simulink model "sensorLib"  (R2020b)
settings: Solver=FixedStepAuto  StartTime=0.0  StopTime=10.0  FixedStep=Ts  RelTol=1e-3
undefined symbols (not defined in the file or in its folder): Sensors, States, Ts
libraries: simulink x3, sharedtransform x1
settings Model: Creator=dbell44  LastModifiedBy=dbell44

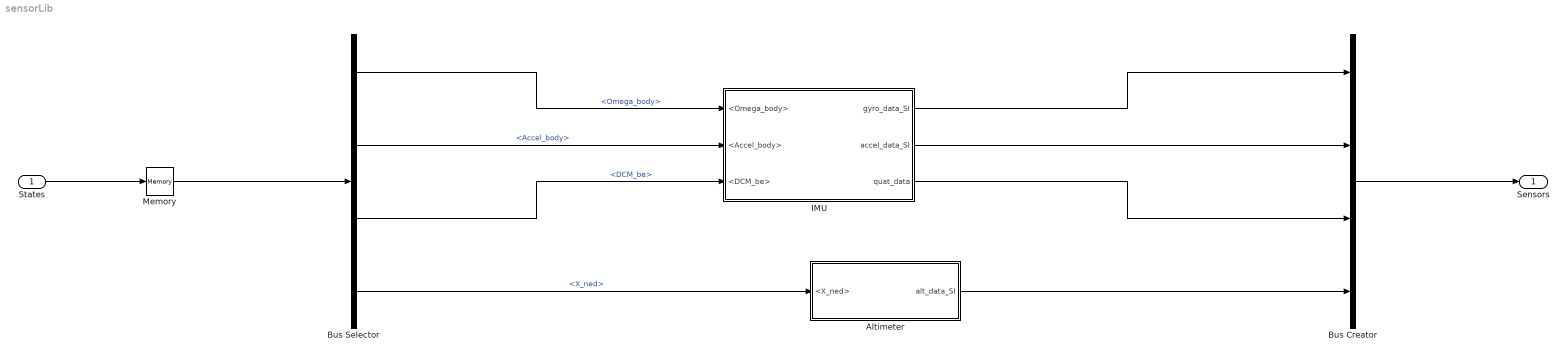
== system sensorLib ==
  States : Inport  OutDataTypeStr=Bus: StatesBus
  Altimeter : Subsystem
  Bus Creator : BusCreator  Inputs=4  OutDataTypeStr=Bus: sensor_data_t
  Bus Selector : BusSelector  OutputSignals=Omega_body,Accel_body,DCM_be,X_ned
  IMU : Subsystem
  Memory : Memory  InitialCondition=States  InheritSampleTime=on
  Sensors : Outport  OutDataTypeStr=Bus: sensor_data_t
  wires:
  States/1 -> Memory/1
  Bus Creator/1 -> Sensors/1
  Memory/1 -> Bus Selector/1
  Bus Selector/1 -> IMU/1(<Omega_body>)  "<Omega_body>"
  Bus Selector/2 -> IMU/2(<Accel_body>)  "<Accel_body>"
  Bus Selector/3 -> IMU/3(<DCM_be>)  "<DCM_be>"
  Bus Selector/4 -> Altimeter/1(<X_ned>)  "<X_ned>"
  Altimeter/1(alt_data_SI) -> Bus Creator/4
  IMU/1(gyro_data_SI) -> Bus Creator/1
  IMU/2(accel_data_SI) -> Bus Creator/2
  IMU/3(quat_data) -> Bus Creator/3

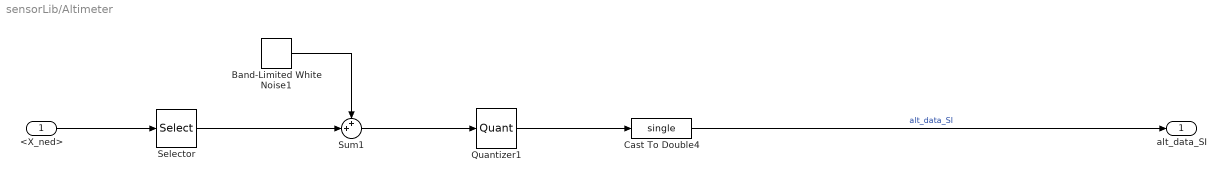
== system sensorLib/Altimeter ==
  <X_ned> : Inport
  Band-Limited White Noise1 : simulink/Sources/Band-Limited White Noise  Cov=Sensors.Altimeter.noiseSpectral  Ts=1/Sensors.Altimeter.Fs  seed=[23341]
  Cast To Double4 : DataTypeConversion  OutDataTypeStr=single
  Quantizer1 : Quantizer  QuantizationInterval=Sensors.Altimeter.Sens  LinearizeAsGain=off
  Selector : Selector  InputPortWidth=3  IndexOptions=Index vector (dialog)  Indices=[3]  OutputSizes=1
  Sum1 : Sum  Inputs=++|
  alt_data_SI : Outport
  wires:
  Cast To Double4/1 -> alt_data_SI/1  "alt_data_SI"
  <X_ned>/1 -> Selector/1
  Selector/1 -> Sum1/2
  Band-Limited White Noise1/1 -> Sum1/1
  Sum1/1 -> Quantizer1/1
  Quantizer1/1 -> Cast To Double4/1

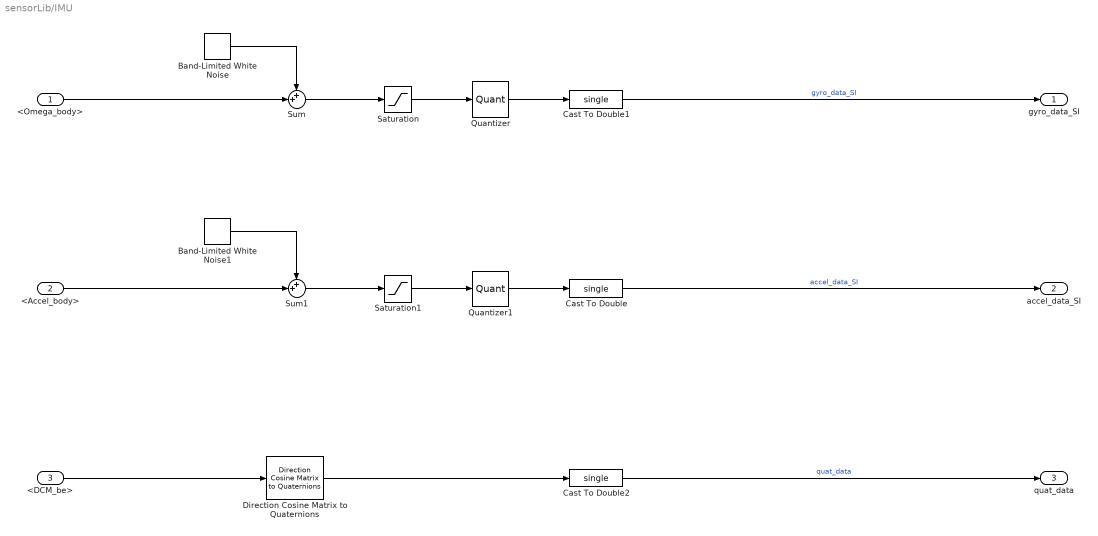
== system sensorLib/IMU ==
  <Omega_body> : Inport
  <Accel_body> : Inport  Port=2
  <DCM_be> : Inport  Port=3
  Band-Limited White Noise : simulink/Sources/Band-Limited White Noise  Cov=Sensors.IMU.Gyro.PSD  Ts=Ts  seed=[23341]
  Band-Limited White Noise1 : simulink/Sources/Band-Limited White Noise  Cov=Sensors.IMU.Accel.PSD  Ts=Ts  seed=[23341]
  Cast To Double : DataTypeConversion  OutDataTypeStr=single
  Cast To Double1 : DataTypeConversion  OutDataTypeStr=single
  Cast To Double2 : DataTypeConversion  OutDataTypeStr=single
  Direction Cosine Matrix to Quaternions : sharedtransform/Direction Cosine Matrix  to Quaternions  aMode=0  action=None  tolerance=eps(2)
      settings: SourceProductBaseCode=AE,PW,MT,UV,VE,VP
  Quantizer : Quantizer  QuantizationInterval=Sensors.IMU.Gyro.Sens  LinearizeAsGain=off
  Quantizer1 : Quantizer  QuantizationInterval=Sensors.IMU.Accel.Sens  LinearizeAsGain=off
  Saturation : Saturate  UpperLimit=Sensors.IMU.Gyro.FSR  LowerLimit=-Sensors.IMU.Gyro.FSR
  Saturation1 : Saturate  UpperLimit=Sensors.IMU.Accel.FSR  LowerLimit=-Sensors.IMU.Gyro.FSR
  Sum : Sum  Inputs=++|
  Sum1 : Sum  Inputs=++|
  gyro_data_SI : Outport
  accel_data_SI : Outport  Port=2
  quat_data : Outport  Port=3
  wires:
  Cast To Double2/1 -> quat_data/1  "quat_data"
  Cast To Double/1 -> accel_data_SI/1  "accel_data_SI"
  Cast To Double1/1 -> gyro_data_SI/1  "gyro_data_SI"
  <Omega_body>/1 -> Sum/2
  Band-Limited White Noise/1 -> Sum/1
  Sum/1 -> Saturation/1
  Saturation/1 -> Quantizer/1
  Quantizer/1 -> Cast To Double1/1
  <Accel_body>/1 -> Sum1/2
  Band-Limited White Noise1/1 -> Sum1/1
  Sum1/1 -> Saturation1/1
  Saturation1/1 -> Quantizer1/1
  Quantizer1/1 -> Cast To Double/1
  <DCM_be>/1 -> Direction Cosine Matrix to Quaternions/1
  Direction Cosine Matrix to Quaternions/1 -> Cast To Double2/1
